simulink model "kk_zad"  (R2021a)
settings: Solver=VariableStepAuto  StartTime=0.0  StopTime=99  RelTol=1e-3
settings Model: Creator=Nina  LastModifiedBy=Nina

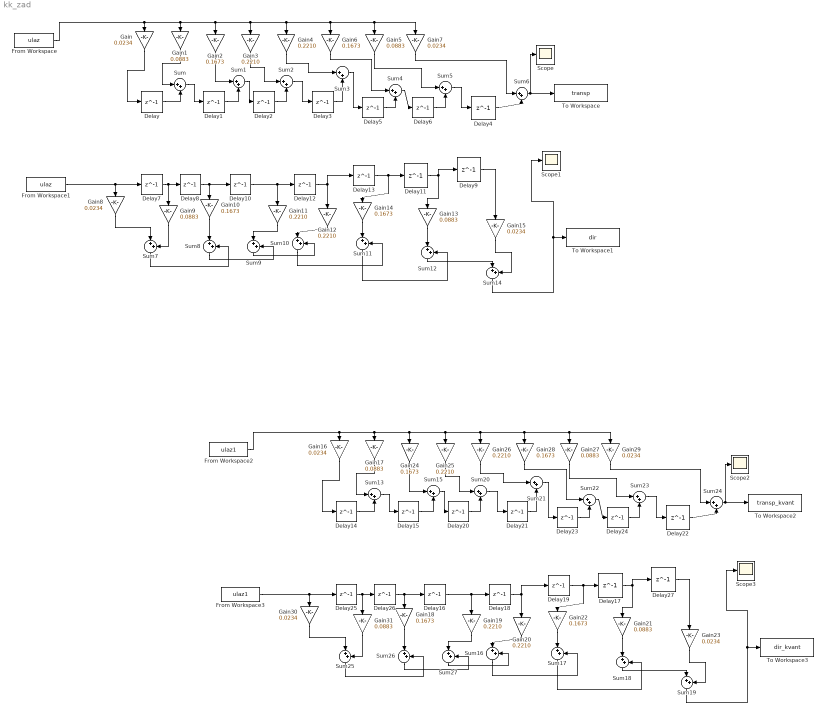
== system kk_zad ==
  Delay{,1..27} (28 alike) : Delay  DelayLength=1  InitialCondition=0  SampleTime=1
  From Workspace : FromWorkspace  VariableName=ulaz
  From Workspace1 : FromWorkspace  VariableName=ulaz
  From Workspace2 : FromWorkspace  VariableName=ulaz1
  From Workspace3 : FromWorkspace  VariableName=ulaz1
  Gain{,7..8,15} (4 alike) : Gain  Gain=0.0234
  Gain{1,5,9,13} (4 alike) : Gain  Gain=0.0883
  Gain{2,6,10,14} (4 alike) : Gain  Gain=0.1673
  Gain{3..4,11..12} (4 alike) : Gain  Gain=0.2210
  Gain{16,23,29..30} (4 alike) : Gain  Gain=0.0234  ParamDataTypeStr=fixdt(1,8,6)
  Gain{17,21,27,31} (4 alike) : Gain  Gain=0.0883  ParamDataTypeStr=fixdt(1,8,6)
  Gain{18,22,24,28} (4 alike) : Gain  Gain=0.1673  ParamDataTypeStr=fixdt(1,8,6)
  Gain{19..20,25..26} (4 alike) : Gain  Gain=0.2210  ParamDataTypeStr=fixdt(1,8,6)
  Scope{,1..3} (4 alike) : Scope
  Sum{,1..27} (28 alike) : Sum  Inputs=|++
  To Workspace : ToWorkspace  VariableName=transp  SampleTime=-1
  To Workspace1 : ToWorkspace  VariableName=dir  SampleTime=-1
  To Workspace2 : ToWorkspace  VariableName=transp_kvant  SampleTime=-1
  To Workspace3 : ToWorkspace  VariableName=dir_kvant  SampleTime=-1
  wires:
  From Workspace/1 -> Gain5/1, Gain7/1, Gain6/1, Gain4/1, Gain3/1, Gain2/1, Gain1/1, Gain/1
  Gain/1 -> Delay/1
  Delay/1 -> Sum/2
  Gain1/1 -> Sum/1
  Sum/1 -> Delay1/1
  Delay1/1 -> Sum1/2
  Gain2/1 -> Sum1/1
  Sum1/1 -> Delay2/1
  Gain3/1 -> Sum2/1
  Delay2/1 -> Sum2/2
  Sum2/1 -> Delay3/1
  Gain4/1 -> Sum3/1
  Delay3/1 -> Sum3/2
  Sum3/1 -> Delay5/1
  Gain6/1 -> Sum4/1
  Delay5/1 -> Sum4/2
  Sum4/1 -> Delay6/1
  Gain5/1 -> Sum5/1
  Delay6/1 -> Sum5/2
  Sum5/1 -> Delay4/1
  Delay4/1 -> Sum6/2
  Gain7/1 -> Sum6/1
  Sum6/1 -> Scope/1, To Workspace/1
  From Workspace1/1 -> Delay7/1, Gain8/1
  Gain8/1 -> Sum7/1
  Delay7/1 -> Delay8/1, Gain9/1
  Gain9/1 -> Sum7/2
  Gain10/1 -> Sum8/1
  Delay8/1 -> Delay10/1, Gain10/1
  Sum7/1 -> Sum8/2
  Delay10/1 -> Delay12/1, Gain11/1
  Sum8/1 -> Sum9/2
  Gain11/1 -> Sum9/1
  Sum9/1 -> Sum10/2
  Gain12/1 -> Sum10/1
  Delay12/1 -> Delay13/1, Gain12/1
  Sum10/1 -> Sum11/2
  Delay13/1 -> Delay11/1, Gain14/1
  Gain14/1 -> Sum11/1
  Sum11/1 -> Sum12/2
  Delay11/1 -> Delay9/1, Gain13/1
  Gain13/1 -> Sum12/1
  Sum12/1 -> Sum14/1
  Delay9/1 -> Gain15/1
  Gain15/1 -> Sum14/2
  Sum14/1 -> Scope1/1, To Workspace1/1
  Gain26/1 -> Sum21/1
  From Workspace2/1 -> Gain27/1, Gain29/1, Gain28/1, Gain26/1, Gain25/1, Gain24/1, Gain17/1, Gain16/1
  Gain24/1 -> Sum15/1
  Delay15/1 -> Sum15/2
  Gain17/1 -> Sum13/1
  Gain25/1 -> Sum20/1
  Sum15/1 -> Delay20/1
  Sum13/1 -> Delay15/1
  Gain30/1 -> Sum25/1
  Sum21/1 -> Delay23/1
  Gain16/1 -> Delay14/1
  Gain29/1 -> Sum24/1
  From Workspace3/1 -> Delay25/1, Gain30/1
  Delay21/1 -> Sum21/2
  Delay16/1 -> Delay18/1, Gain19/1
  Delay26/1 -> Delay16/1, Gain18/1
  Sum27/1 -> Sum16/2
  Sum25/1 -> Sum26/2
  Sum23/1 -> Delay22/1
  Gain20/1 -> Sum16/1
  Gain27/1 -> Sum23/1
  Delay24/1 -> Sum23/2
  Delay22/1 -> Sum24/2
  Sum20/1 -> Delay21/1
  Delay18/1 -> Delay19/1, Gain20/1
  Delay19/1 -> Delay17/1, Gain22/1
  Gain31/1 -> Sum25/2
  Gain28/1 -> Sum22/1
  Sum24/1 -> Scope2/1, To Workspace2/1
  Sum22/1 -> Delay24/1
  Delay27/1 -> Gain23/1
  Sum18/1 -> Sum19/1
  Delay20/1 -> Sum20/2
  Sum16/1 -> Sum17/2
  Delay14/1 -> Sum13/2
  Delay17/1 -> Delay27/1, Gain21/1
  Delay25/1 -> Delay26/1, Gain31/1
  Sum19/1 -> Scope3/1, To Workspace3/1
  Sum26/1 -> Sum27/2
  Gain18/1 -> Sum26/1
  Delay23/1 -> Sum22/2
  Gain23/1 -> Sum19/2
  Sum17/1 -> Sum18/2
  Gain19/1 -> Sum27/1
  Gain22/1 -> Sum17/1
  Gain21/1 -> Sum18/1
